simulink model "RefModel_AeroDyn_Sim2"  (R2019b)
settings: Solver=ode1  StartTime=tspan(1)  StopTime=inf  FixedStep=1/sensorFs.imuUpdateFs  RelTol=1e-3  EnableMultiTasking=on
undefined symbols (not defined in the file or in its folder): ACTUATOR_SET, Earth, ENVIRONMENT_SET, F, Light, MIL, sensorFs, SIM_SENSOR_SET, UAVPARAM_SET, WGS84
libraries: simulink x10, aerolibactuator x9, aerolibnav x6, sharedutil x5, shared6dofsys x3, aerolibwind2 x2, aerolibasang x2, aerolibatmos2 x1, aerolibconvert2 x1, aerolibgravity2 x1, aerolibtransform2 x1
(part 3 of 3)

== system RefModel_AeroDyn_Sim2/Sensor Model (noise)/Ublox1/add noise1 ==
  noise_flag : Inport
  signal : Inport  Port=2
  Add : Sum
  Add1 : Sum
  Divide : Product  Inputs=**
  Divide1 : Product  Inputs=**
  Divide2 : Product  Inputs=**
  MATLAB Function : MATLAB Function  TreatAsAtomicUnit=on
  Random Number : RandomNumber  Seed=[18,19,20]
  bias : Constant  Value=[0,0,0]
  bias1 : Constant  Value=SIM_SENSOR_SET.Ublox1.std_lla
  Out1 : Outport
  wires:
  bias1/1 -> Divide1/1
  bias/1 -> Add/1
  Divide/1 -> Add/2
  Random Number/1 -> Divide/1
  Divide1/1 -> Divide/2
  MATLAB Function/1(k) -> Divide1/2
  signal/1 -> MATLAB Function/1(u), Add1/2
  noise_flag/1 -> Divide2/1
  Divide2/1 -> Add1/1
  Add/1 -> Divide2/2
  Add1/1 -> Out1/1

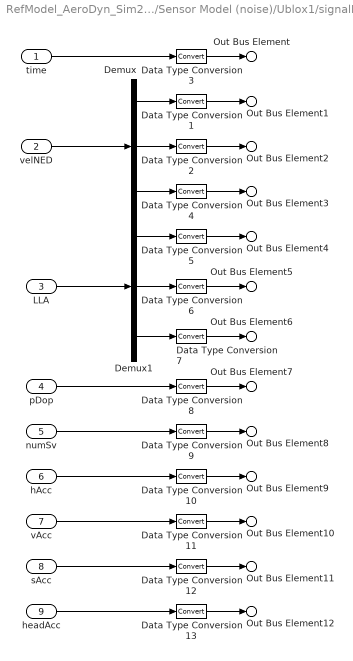
== system RefModel_AeroDyn_Sim2/Sensor Model (noise)/Ublox1/signalBus ==
  time : Inport
  velNED : Inport  Port=2
  LLA : Inport  Port=3
  pDop : Inport  Port=4
  numSv : Inport  Port=5
  hAcc : Inport  Port=6
  vAcc : Inport  Port=7
  sAcc : Inport  Port=8
  headAcc : Inport  Port=9
  Data Type Conversion{1..13} (13 alike) : DataTypeConversion
  Demux : Demux  Outputs=3
  Demux1 : Demux  Outputs=3
  Out Bus Element : Outport  PortName=bus  Element=time
  Out Bus Element1 : Outport  PortName=bus  Element=velN
  Out Bus Element2 : Outport  PortName=bus  Element=velE
  Out Bus Element3 : Outport  PortName=bus  Element=velD
  Out Bus Element4 : Outport  PortName=bus  Element=Lat
  Out Bus Element5 : Outport  PortName=bus  Element=Lon
  Out Bus Element6 : Outport  PortName=bus  Element=height
  Out Bus Element7 : Outport  PortName=bus  Element=pDop
  Out Bus Element8 : Outport  PortName=bus  Element=numSv
  Out Bus Element9 : Outport  PortName=bus  Element=hAcc
  Out Bus Element10 : Outport  PortName=bus  Element=vAcc
  Out Bus Element11 : Outport  PortName=bus  Element=sAcc
  Out Bus Element12 : Outport  PortName=bus  Element=headAcc
  wires:
  Demux/3 -> Data Type Conversion4/1
  Demux/2 -> Data Type Conversion2/1
  time/1 -> Data Type Conversion3/1
  Demux/1 -> Data Type Conversion1/1
  Demux1/1 -> Data Type Conversion5/1
  Demux1/2 -> Data Type Conversion6/1
  Demux1/3 -> Data Type Conversion7/1
  numSv/1 -> Data Type Conversion9/1
  pDop/1 -> Data Type Conversion8/1
  velNED/1 -> Demux/1
  LLA/1 -> Demux1/1
  Data Type Conversion3/1 -> Out Bus Element/1
  Data Type Conversion1/1 -> Out Bus Element1/1
  Data Type Conversion2/1 -> Out Bus Element2/1
  Data Type Conversion4/1 -> Out Bus Element3/1
  Data Type Conversion5/1 -> Out Bus Element4/1
  Data Type Conversion6/1 -> Out Bus Element5/1
  Data Type Conversion7/1 -> Out Bus Element6/1
  Data Type Conversion8/1 -> Out Bus Element7/1
  Data Type Conversion9/1 -> Out Bus Element8/1
  Data Type Conversion10/1 -> Out Bus Element9/1
  hAcc/1 -> Data Type Conversion10/1
  vAcc/1 -> Data Type Conversion11/1
  Data Type Conversion11/1 -> Out Bus Element10/1
  Data Type Conversion12/1 -> Out Bus Element11/1
  sAcc/1 -> Data Type Conversion12/1
  headAcc/1 -> Data Type Conversion13/1
  Data Type Conversion13/1 -> Out Bus Element12/1

== system RefModel_AeroDyn_Sim2/Sensor Model (noise)/um482/Subsystem ==
  Inport : Inport
  Inport1 : Inport  Port=2
  Demux7 : Demux  Outputs=3
  Demux8 : Demux  Outputs=3
  Mux : Mux  Inputs=2
  Mux1 : Mux  Inputs=2
  Mux2 : Mux  Inputs=2
  Outport : Outport
  Outport1 : Outport  Port=2
  Outport2 : Outport  Port=3
  wires:
  Demux7/1 -> Mux/1  "yaw [deg]"
  Demux8/1 -> Mux/2  "yaw [deg]"
  Inport/1 -> Demux7/1
  Mux/1 -> Outport/1
  Demux8/3 -> Mux2/2  "roll [deg]"
  Demux7/2 -> Mux1/1
  Inport1/1 -> Demux8/1
  Mux2/1 -> Outport2/1
  Mux1/1 -> Outport1/1
  Demux8/2 -> Mux1/2  "pitch [deg]"
  Demux7/3 -> Mux2/1  "roll [deg]"

== system RefModel_AeroDyn_Sim2/Sensor Model (noise)/um482/Subsystem1 ==
  Inport : Inport
  Inport1 : Inport  Port=2
  Demux7 : Demux  Outputs=3
  Demux8 : Demux  Outputs=3
  Mux : Mux  Inputs=2
  Mux1 : Mux  Inputs=2
  Mux2 : Mux  Inputs=2
  Outport : Outport
  Outport1 : Outport  Port=2
  Outport2 : Outport  Port=3
  wires:
  Demux7/3 -> Mux2/1  "roll [deg]"
  Demux8/2 -> Mux1/2  "pitch [deg]"
  Mux1/1 -> Outport1/1
  Mux2/1 -> Outport2/1
  Inport1/1 -> Demux8/1
  Demux7/2 -> Mux1/1
  Demux8/3 -> Mux2/2  "roll [deg]"
  Mux/1 -> Outport/1
  Inport/1 -> Demux7/1
  Demux8/1 -> Mux/2  "yaw [deg]"
  Demux7/1 -> Mux/1  "yaw [deg]"

== system RefModel_AeroDyn_Sim2/Sensor Model (noise)/um482/Subsystem2 ==
  In : Inport
  Compare To Zero : simulink/Logic and Bit Operations/Compare To Zero  relop===  OutDataTypeStr=boolean
  Constant : Constant  Value=1/sample_freq
  Digital Clock : DigitalClock  SampleTime=1/sensorFs.imuUpdateFs
  Math Function : Math  Operator=rem  SignedPower=off  SaturateOnIntegerOverflow=on
  Scope1 : Scope
  Subsystem : Subsystem
  zeroHold : Outport
  wires:
  Digital Clock/1 -> Math Function/1
  Constant/1 -> Math Function/2
  Math Function/1 -> Compare To Zero/1
  Compare To Zero/1 -> Scope1/1, Subsystem/Enable
  Subsystem/1(Out1) -> zeroHold/1
  In/1 -> Subsystem/1(In1)

== system RefModel_AeroDyn_Sim2/Sensor Model (noise)/um482/add noise ==
  noise_flag : Inport
  signal : Inport  Port=2
  Add : Sum
  Add1 : Sum
  Divide : Product  Inputs=**
  Divide1 : Product  Inputs=**
  Random Number : RandomNumber  Seed=[18,19,20]
  bias : Constant  Value=[0,0,0]
  bias1 : Constant  Value=SIM_SENSOR_SET.um482.std_gpsvel
  Out1 : Outport
  wires:
  signal/1 -> Add1/2
  Random Number/1 -> Divide/1
  Divide/1 -> Add/2
  bias/1 -> Add/1
  bias1/1 -> Divide/2
  Add/1 -> Divide1/2
  Divide1/1 -> Add1/1
  noise_flag/1 -> Divide1/1
  Add1/1 -> Out1/1

== system RefModel_AeroDyn_Sim2/Sensor Model (noise)/um482/add noise1 ==
  noise_flag : Inport
  signal : Inport  Port=2
  Add : Sum
  Add1 : Sum
  Divide : Product  Inputs=**
  Divide1 : Product  Inputs=**
  Divide2 : Product  Inputs=**
  MATLAB Function : MATLAB Function  TreatAsAtomicUnit=on
  Random Number : RandomNumber  Seed=[18,19,20]
  bias : Constant  Value=[0,0,0]
  bias1 : Constant  Value=SIM_SENSOR_SET.um482.std_lla
  Out1 : Outport
  wires:
  bias1/1 -> Divide1/1
  bias/1 -> Add/1
  Divide/1 -> Add/2
  Random Number/1 -> Divide/1
  Divide1/1 -> Divide/2
  MATLAB Function/1(k) -> Divide1/2
  signal/1 -> MATLAB Function/1(u), Add1/2
  noise_flag/1 -> Divide2/1
  Divide2/1 -> Add1/1
  Add/1 -> Divide2/2
  Add1/1 -> Out1/1

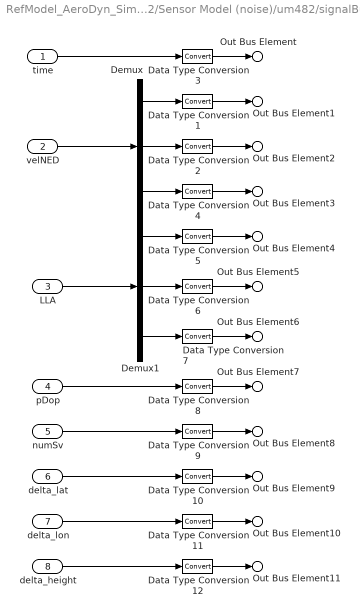
== system RefModel_AeroDyn_Sim2/Sensor Model (noise)/um482/signalBus ==
  time : Inport
  velNED : Inport  Port=2
  LLA : Inport  Port=3
  pDop : Inport  Port=4
  numSv : Inport  Port=5
  delta_lat : Inport  Port=6
  delta_lon : Inport  Port=7
  delta_height : Inport  Port=8
  Data Type Conversion{1..12} (12 alike) : DataTypeConversion
  Demux : Demux  Outputs=3
  Demux1 : Demux  Outputs=3
  Out Bus Element : Outport  PortName=bus  Element=time
  Out Bus Element1 : Outport  PortName=bus  Element=velN
  Out Bus Element2 : Outport  PortName=bus  Element=velE
  Out Bus Element3 : Outport  PortName=bus  Element=velD
  Out Bus Element4 : Outport  PortName=bus  Element=Lat
  Out Bus Element5 : Outport  PortName=bus  Element=Lon
  Out Bus Element6 : Outport  PortName=bus  Element=height
  Out Bus Element7 : Outport  PortName=bus  Element=pDop
  Out Bus Element8 : Outport  PortName=bus  Element=numSv
  Out Bus Element9 : Outport  PortName=bus  Element=delta_lat
  Out Bus Element10 : Outport  PortName=bus  Element=delta_lon
  Out Bus Element11 : Outport  PortName=bus  Element=delta_height
  wires:
  Demux/3 -> Data Type Conversion4/1
  Demux/2 -> Data Type Conversion2/1
  time/1 -> Data Type Conversion3/1
  Demux/1 -> Data Type Conversion1/1
  Demux1/1 -> Data Type Conversion5/1
  Demux1/2 -> Data Type Conversion6/1
  Demux1/3 -> Data Type Conversion7/1
  numSv/1 -> Data Type Conversion9/1
  pDop/1 -> Data Type Conversion8/1
  velNED/1 -> Demux/1
  LLA/1 -> Demux1/1
  Data Type Conversion3/1 -> Out Bus Element/1
  Data Type Conversion1/1 -> Out Bus Element1/1
  Data Type Conversion2/1 -> Out Bus Element2/1
  Data Type Conversion4/1 -> Out Bus Element3/1
  Data Type Conversion5/1 -> Out Bus Element4/1
  Data Type Conversion6/1 -> Out Bus Element5/1
  Data Type Conversion7/1 -> Out Bus Element6/1
  Data Type Conversion8/1 -> Out Bus Element7/1
  Data Type Conversion9/1 -> Out Bus Element8/1
  Data Type Conversion10/1 -> Out Bus Element9/1
  delta_lat/1 -> Data Type Conversion10/1
  delta_lon/1 -> Data Type Conversion11/1
  Data Type Conversion11/1 -> Out Bus Element10/1
  Data Type Conversion12/1 -> Out Bus Element11/1
  delta_height/1 -> Data Type Conversion12/1

== system RefModel_AeroDyn_Sim2/UAV Dynamics/6DOF (Quaternion)/Velocity Conversion ==
  in : Inport  Unit=m/s
  Unit Conversion : UnitConversion
  out : Outport  VectorParamsAs1DForOutWhenUnconnected=off
  wires:
  Unit Conversion/1 -> out/1
  in/1 -> Unit Conversion/1

== system RefModel_AeroDyn_Sim2/UAV Dynamics/6DOF (Quaternion)/Velocity Conversion1 ==
  in : Inport  Unit=m/s
  Unit Conversion : UnitConversion
  out : Outport  VectorParamsAs1DForOutWhenUnconnected=off
  wires:
  Unit Conversion/1 -> out/1
  in/1 -> Unit Conversion/1

== system RefModel_AeroDyn_Sim2/UAV Dynamics/6DOF (Quaternion)/Velocity Conversion2 ==
  in : Inport  Unit=m/s
  Unit Conversion : UnitConversion
  out : Outport  Unit=m/s  VectorParamsAs1DForOutWhenUnconnected=off
  wires:
  Unit Conversion/1 -> out/1
  in/1 -> Unit Conversion/1

== system RefModel_AeroDyn_Sim2/UAV Dynamics/6DOF (Quaternion)/transform to Inertial axes  ==
  x y z : Inport
  transform coefficients : Inport  Port=2
  Product : Product  Multiplication=Matrix(*)  SaturateOnIntegerOverflow=on  InputSameDT=on  OutDataTypeStr=Inherit: Same as first input
  Reshape1 : Reshape  OutputDimensionality=Column vector (2-D)
  Reshape2 : Reshape
  Ve : Outport  VectorParamsAs1DForOutWhenUnconnected=off
  wires:
  Reshape2/1 -> Ve/1
  Reshape1/1 -> Product/2
  x y z/1 -> Reshape1/1
  transform coefficients/1 -> Product/1
  Product/1 -> Reshape2/1

== system RefModel_AeroDyn_Sim2/Force and Moment/Aero Surface/Lateral Channel/CY ==
  beta : Inport
  rudder : Inport  Port=2
  airspeed : Inport  Port=3
  CYDr : Constant  Value=UAVPARAM_SET.AeroParam.CY_rudder
      settings: AttributesFormatString=%<Value>
  CYb : Constant  Value=UAVPARAM_SET.AeroParam.CY_beta
      settings: AttributesFormatString=%<Value>
  Product : Product  SaturateOnIntegerOverflow=on  OutDataTypeStr=Inherit: Same as first input
  Product1 : Product  SaturateOnIntegerOverflow=on  OutDataTypeStr=Inherit: Same as first input
  Sum2 : Sum  SaturateOnIntegerOverflow=on
  CY : Outport  VectorParamsAs1DForOutWhenUnconnected=off
  wires:
  Product1/1 -> Sum2/2
  rudder/1 -> Product1/2
  CYDr/1 -> Product1/1
  Product/1 -> Sum2/1
  Sum2/1 -> CY/1
  beta/1 -> Product/2
  CYb/1 -> Product/1

== system RefModel_AeroDyn_Sim2/Force and Moment/Aero Surface/Lateral Channel/Cl ==
  beta : Inport
  aileron : Inport  Port=2
  rudder : Inport  Port=3
  p,q,r : Inport  Port=4
  Airspeed : Inport  Port=5
  wingspan : Inport  Port=6
  ClDa : Constant  Value=UAVPARAM_SET.AeroParam.Cl_aileron
      settings: AttributesFormatString=%<Value>
  ClDr : Constant  Value=UAVPARAM_SET.AeroParam.Cl_rudder
      settings: AttributesFormatString=%<Value>
  Clb : Constant  Value=UAVPARAM_SET.AeroParam.Cl_beta
      settings: AttributesFormatString=%<Value>
  Product1 : Product  SaturateOnIntegerOverflow=on  OutDataTypeStr=Inherit: Same as first input
  Product4 : Product  SaturateOnIntegerOverflow=on  OutDataTypeStr=Inherit: Same as first input
  Product5 : Product  SaturateOnIntegerOverflow=on  OutDataTypeStr=Inherit: Same as first input
  Sum : Sum  Inputs=+++++  SaturateOnIntegerOverflow=on
  roll factors : Subsystem
  Cl : Outport  VectorParamsAs1DForOutWhenUnconnected=off
  wires:
  roll factors/1(Clp) -> Sum/4
  Product5/1 -> Sum/2  "CldA"
  Airspeed/1 -> roll factors/2(Airspeed)
  p,q,r/1 -> roll factors/1(p,q,r)
  roll factors/2(Clr) -> Sum/5
  Product1/1 -> Sum/3  "Cldr"
  Product4/1 -> Sum/1  "Clb"
  Sum/1 -> Cl/1
  rudder/1 -> Product1/2
  ClDr/1 -> Product1/1
  aileron/1 -> Product5/2
  ClDa/1 -> Product5/1
  beta/1 -> Product4/2
  Clb/1 -> Product4/1
  wingspan/1 -> roll factors/3(wingspan)

== system RefModel_AeroDyn_Sim2/Force and Moment/Aero Surface/Lateral Channel/Cn ==
  beta : Inport
  aileron : Inport  Port=2
  rudder : Inport  Port=3
  p,q,r : Inport  Port=4
  Airspeed : Inport  Port=5
  wingspan : Inport  Port=6
  CnDa : Constant  Value=UAVPARAM_SET.AeroParam.Cn_aileron
      settings: AttributesFormatString=%<Value>
  CnDr : Constant  Value=UAVPARAM_SET.AeroParam.Cn_rudder
      settings: AttributesFormatString=%<Value>
  Cnb : Constant  Value=UAVPARAM_SET.AeroParam.Cn_beta
      settings: AttributesFormatString=%<Value>
  Product1 : Product  SaturateOnIntegerOverflow=on  OutDataTypeStr=Inherit: Same as first input
  Product4 : Product  SaturateOnIntegerOverflow=on  OutDataTypeStr=Inherit: Same as first input
  Product5 : Product  SaturateOnIntegerOverflow=on  OutDataTypeStr=Inherit: Same as first input
  Sum : Sum  Inputs=+++++  SaturateOnIntegerOverflow=on
  yaw factors : Subsystem
  Cn : Outport  VectorParamsAs1DForOutWhenUnconnected=off
  wires:
  Airspeed/1 -> yaw factors/2(Airspeed)
  p,q,r/1 -> yaw factors/1(p,q,r)
  Cnb/1 -> Product4/1
  beta/1 -> Product4/2
  CnDa/1 -> Product5/1
  Product5/1 -> Sum/2
  aileron/1 -> Product5/2
  CnDr/1 -> Product1/1
  rudder/1 -> Product1/2
  Sum/1 -> Cn/1
  Product1/1 -> Sum/3
  yaw factors/2(Cnr) -> Sum/5
  yaw factors/1(Cnp) -> Sum/4
  Product4/1 -> Sum/1
  wingspan/1 -> yaw factors/3(wingspan)

== system RefModel_AeroDyn_Sim2/Force and Moment/Aero Surface/Longitudinal Channel/CD ==
  alpha : Inport
  airspeed : Inport  Port=2
  Apolar (A2) : Constant  Value=UAVPARAM_SET.AeroParam.CD_alpha
      settings: AttributesFormatString=%<Value>
  CD0 : Constant  Value=UAVPARAM_SET.AeroParam.CD0
      settings: AttributesFormatString=%<Value>
  Gain : Gain  Gain=-1  SaturateOnIntegerOverflow=on  OutDataTypeStr=Inherit: Same as input  ParamDataTypeStr=Inherit: Same as input
      settings: AttributesFormatString=%<Gain>
  Product : Product  SaturateOnIntegerOverflow=on  OutDataTypeStr=Inherit: Same as first input
  Sum1 : Sum  Inputs=|++  SaturateOnIntegerOverflow=on
  CD : Outport  VectorParamsAs1DForOutWhenUnconnected=off
  wires:
  Gain/1 -> CD/1
  Apolar (A2)/1 -> Product/1
  alpha/1 -> Product/2
  Sum1/1 -> Gain/1
  Product/1 -> Sum1/1
  CD0/1 -> Sum1/2

== system RefModel_AeroDyn_Sim2/Force and Moment/Aero Surface/Longitudinal Channel/CL ==
  alpha : Inport
  elevator : Inport  Port=2
  airspeed : Inport  Port=3
  CL0 : Constant  Value=UAVPARAM_SET.AeroParam.CL0
      settings: AttributesFormatString=%<Value>
  CLDe : Constant  Value=UAVPARAM_SET.AeroParam.CL_elevator
      settings: AttributesFormatString=%<Value>
  CLa : Constant  Value=UAVPARAM_SET.AeroParam.CL_alpha
      settings: AttributesFormatString=%<Value>
  Product1 : Product  SaturateOnIntegerOverflow=on  OutDataTypeStr=Inherit: Same as first input
  Product4 : Product  SaturateOnIntegerOverflow=on  OutDataTypeStr=Inherit: Same as first input
  Sum : Sum  Inputs=++++  SaturateOnIntegerOverflow=on
  Y-down : Gain  Gain=-1  SaturateOnIntegerOverflow=on  OutDataTypeStr=Inherit: Same as input  ParamDataTypeStr=Inherit: Same as input
      settings: AttributesFormatString=%<Gain>
  CL : Outport  VectorParamsAs1DForOutWhenUnconnected=off
  wires:
  CL0/1 -> Sum/1
  Product1/1 -> Sum/3
  Sum/1 -> Y-down/1
  elevator/1 -> Product1/2
  CLDe/1 -> Product1/1
  alpha/1 -> Product4/2
  CLa/1 -> Product4/1
  Product4/1 -> Sum/2
  Y-down/1 -> CL/1  "CL"

== system RefModel_AeroDyn_Sim2/Force and Moment/Aero Surface/Longitudinal Channel/Cm ==
  alpha : Inport
  De : Inport  Port=2
  p,q,r : Inport  Port=3
  airspeed : Inport  Port=4
  Cm0 : Constant  Value=UAVPARAM_SET.AeroParam.Cm0
      settings: AttributesFormatString=%<Value>
  CmDe : Constant  Value=UAVPARAM_SET.AeroParam.Cm_elevator
      settings: AttributesFormatString=%<Value>
  Cma : Constant  Value=UAVPARAM_SET.AeroParam.Cm_alpha
      settings: AttributesFormatString=%<Value>
  Cma1 : Constant  Value=UAVPARAM_SET.AeroParam.Cm_q
      settings: AttributesFormatString=%<Value>
  Get q : Selector  InputPortWidth=3  IndexOptions=Index vector (dialog)  Indices=2  OutputSizes=[(-2)]
  Product1 : Product  SaturateOnIntegerOverflow=on  OutDataTypeStr=Inherit: Same as first input
  Product3 : Product  SaturateOnIntegerOverflow=on  OutDataTypeStr=Inherit: Same as first input
  Product4 : Product  SaturateOnIntegerOverflow=on  OutDataTypeStr=Inherit: Same as first input
  Sum : Sum  Inputs=+++++  SaturateOnIntegerOverflow=on
  Cm : Outport  VectorParamsAs1DForOutWhenUnconnected=off
  wires:
  Get q/1 -> Product3/2
  Product3/1 -> Sum/5  "cmq"
  p,q,r/1 -> Get q/1
  Cma1/1 -> Product3/1
  Product1/1 -> Sum/3  "cmde"
  Product4/1 -> Sum/2  "cma"
  Sum/1 -> Cm/1  "total"
  De/1 -> Product1/2
  CmDe/1 -> Product1/1
  alpha/1 -> Product4/2
  Cma/1 -> Product4/1
  Cm0/1 -> Sum/1  "cm0"

== system RefModel_AeroDyn_Sim2/Force and Moment/Rotor Force/Left Back/Rotor 2814 ==
  pwm : Inport
  Constant : Constant  Value=ACTUATOR_SET.tiltRotor.poly_fromPwmTopull
  Constant1 : Constant  Value=ACTUATOR_SET.tiltRotor.poly_fromPwmToTorque
  Constant2 : Constant  Value=[0,0]
  Constant3 : Constant  Value=ACTUATOR_SET.tiltRotorLeft.torqueSign
  Divide : Product  Inputs=**
  MATLAB Function : MATLAB Function  TreatAsAtomicUnit=on
  MATLAB Function1 : MATLAB Function  TreatAsAtomicUnit=on
  Mux : Mux  Inputs=2
  pull : Outport
  torque : Outport  Port=2
  wires:
  pwm/1 -> MATLAB Function1/1(u), MATLAB Function/1(u)
  MATLAB Function/1(y) -> pull/1
  Constant/1 -> MATLAB Function/2(poly)
  Constant1/1 -> MATLAB Function1/2(poly)
  MATLAB Function1/1(y) -> Divide/1
  Constant3/1 -> Divide/2
  Divide/1 -> Mux/2
  Constant2/1 -> Mux/1
  Mux/1 -> torque/1

== system RefModel_AeroDyn_Sim2/Force and Moment/Rotor Force/Left Forward/Rotor 5208 ==
  pwm : Inport
  Constant : Constant  Value=ACTUATOR_SET.verticalRotor.poly_fromPwmTopull
  Constant1 : Constant  Value=ACTUATOR_SET.verticalRotor.poly_fromPwmToTorque
  Constant2 : Constant  Value=[0,0]
  Constant3 : Constant  Value=ACTUATOR_SET.verticalRotorLeft.torqueSign
  Divide : Product  Inputs=**
  MATLAB Function : MATLAB Function  TreatAsAtomicUnit=on
  MATLAB Function1 : MATLAB Function  TreatAsAtomicUnit=on
  Mux : Mux  Inputs=2
  pull : Outport
  torque : Outport  Port=2
  wires:
  Constant1/1 -> MATLAB Function1/2(poly)
  Constant/1 -> MATLAB Function/2(poly)
  MATLAB Function/1(y) -> pull/1
  pwm/1 -> MATLAB Function/1(u), MATLAB Function1/1(u)
  Constant2/1 -> Mux/1
  Mux/1 -> torque/1
  Constant3/1 -> Divide/2
  MATLAB Function1/1(y) -> Divide/1
  Divide/1 -> Mux/2

== system RefModel_AeroDyn_Sim2/Force and Moment/Rotor Force/Right Back/Rotor 2814 ==
  pwm : Inport
  Constant : Constant  Value=ACTUATOR_SET.tiltRotor.poly_fromPwmTopull
  Constant1 : Constant  Value=ACTUATOR_SET.tiltRotor.poly_fromPwmToTorque
  Constant2 : Constant  Value=[0,0]
  Constant3 : Constant  Value=ACTUATOR_SET.tiltRotorRight.torqueSign
  Divide : Product  Inputs=**
  MATLAB Function : MATLAB Function  TreatAsAtomicUnit=on
  MATLAB Function1 : MATLAB Function  TreatAsAtomicUnit=on
  Mux : Mux  Inputs=2
  pull : Outport
  torque : Outport  Port=2
  wires:
  pwm/1 -> MATLAB Function1/1(u), MATLAB Function/1(u)
  MATLAB Function/1(y) -> pull/1
  Constant/1 -> MATLAB Function/2(poly)
  Constant1/1 -> MATLAB Function1/2(poly)
  Constant2/1 -> Mux/1
  Constant3/1 -> Divide/2
  Divide/1 -> Mux/2
  Mux/1 -> torque/1
  MATLAB Function1/1(y) -> Divide/1

== system RefModel_AeroDyn_Sim2/Force and Moment/Rotor Force/Right Forward/Rotor 5208 ==
  pwm : Inport
  Constant : Constant  Value=ACTUATOR_SET.verticalRotor.poly_fromPwmTopull
  Constant1 : Constant  Value=ACTUATOR_SET.verticalRotor.poly_fromPwmToTorque
  Constant2 : Constant  Value=[0,0]
  Constant3 : Constant  Value=ACTUATOR_SET.verticalRotorRight.torqueSign
  Divide : Product  Inputs=**
  MATLAB Function : MATLAB Function  TreatAsAtomicUnit=on
  MATLAB Function1 : MATLAB Function  TreatAsAtomicUnit=on
  Mux : Mux  Inputs=2
  pull : Outport
  torque : Outport  Port=2
  wires:
  Constant1/1 -> MATLAB Function1/2(poly)
  Constant/1 -> MATLAB Function/2(poly)
  MATLAB Function/1(y) -> pull/1
  pwm/1 -> MATLAB Function1/1(u), MATLAB Function/1(u)
  Constant2/1 -> Mux/1
  Mux/1 -> torque/1
  MATLAB Function1/1(y) -> Divide/1
  Divide/1 -> Mux/2
  Constant3/1 -> Divide/2

== system RefModel_AeroDyn_Sim2/Sensor Model (noise)/Airspeed1/Subsystem3/Subsystem ==
  In1 : Inport
  Enable : EnablePort
  Out1 : Outport
  wires:
  In1/1 -> Out1/1

== system RefModel_AeroDyn_Sim2/Sensor Model (noise)/Baro1/Subsystem3/Subsystem ==
  In1 : Inport
  Enable : EnablePort
  Out1 : Outport
  wires:
  In1/1 -> Out1/1

== system RefModel_AeroDyn_Sim2/Sensor Model (noise)/IMU1/Subsystem2/Subsystem ==
  In1 : Inport
  Enable : EnablePort
  Out1 : Outport
  wires:
  In1/1 -> Out1/1

== system RefModel_AeroDyn_Sim2/Sensor Model (noise)/IMU1/Subsystem3/NOISE ==
  In1 : Inport
  In2 : Inport  Port=2
  In3 : Inport  Port=3
  In4 : Inport  Port=4
  In5 : Inport  Port=5
  Action Port : ActionPort  ActionPortLabel=case [ 1 ]:
  Three-axis Inertial Measurement Unit : aerolibnav/Three-axis Inertial Measurement Unit  units=Metric (MKS)  imu=[0 0 0]  i_Ts=1/sensorFs.imuUpdateFs  dtype_a=off  w_a=190  z_a=0.707  a_sf_cc=[1 0 0; 0 1 0; 0 0 1]  a_bias=SIM_SENSOR_SET.IMU1.acc_bias  a_sat="[-inf  -inf  -inf  inf inf inf]"  dtype_g=off  w_g=190  z_g=0.707  g_sf_cc=[1 0 0; 0 1 0; 0 0 1]  g_bias=SIM_SENSOR_SET.IMU1.gyro_bias  g_sens=[0 0 0]  g_sat="[-inf  -inf  -inf  inf inf inf]"  i_rand=on  i_seeds=[23093 23094 23095 23096 23097 23098]  i_pow=[SIM_SENSOR_SET.IMU1.S_acc, SIM_SENSOR_SET.IMU1.S_gyro]
  accel : Outport
  Out2 : Outport  Port=2
  wires:
  In1/1 -> Three-axis Inertial Measurement Unit/1
  In2/1 -> Three-axis Inertial Measurement Unit/2
  Three-axis Inertial Measurement Unit/2 -> Out2/1
  Three-axis Inertial Measurement Unit/1 -> accel/1  "accel"
  In5/1 -> Three-axis Inertial Measurement Unit/5
  In3/1 -> Three-axis Inertial Measurement Unit/3
  In4/1 -> Three-axis Inertial Measurement Unit/4

== system RefModel_AeroDyn_Sim2/Sensor Model (noise)/IMU1/Subsystem3/NOISE FREE ==
  In1 : Inport
  In2 : Inport  Port=2
  In3 : Inport  Port=3
  In4 : Inport  Port=4
  In5 : Inport  Port=5
  Action Port : ActionPort  ActionPortLabel=default:
  Three-axis Inertial Measurement Unit1 : aerolibnav/Three-axis Inertial Measurement Unit  units=Metric (MKS)  imu=[0 0 0]  i_Ts=1/sensorFs.imuUpdateFs  dtype_a=off  w_a=190  z_a=0.707  a_sf_cc=[1 0 0; 0 1 0; 0 0 1]  a_bias=[0,0,0]  a_sat="[-inf  -inf  -inf  inf inf inf]"  dtype_g=off  w_g=190  z_g=0.707  g_sf_cc=[1 0 0; 0 1 0; 0 0 1]  g_bias=[0 0 0]  g_sens=[0 0 0]  g_sat="[-inf  -inf  -inf  inf inf inf]"  i_rand=off  i_seeds=[23093 23094 23095 23096 23097 23098]  i_pow=[SIM_SENSOR_SET.IMU1.S_acc, SIM_SENSOR_SET.IMU1.S_gyro]
  accel : Outport
  Out2 : Outport  Port=2
  wires:
  In2/1 -> Three-axis Inertial Measurement Unit1/2
  In1/1 -> Three-axis Inertial Measurement Unit1/1
  In5/1 -> Three-axis Inertial Measurement Unit1/5
  Three-axis Inertial Measurement Unit1/1 -> accel/1  "accel"
  In3/1 -> Three-axis Inertial Measurement Unit1/3
  In4/1 -> Three-axis Inertial Measurement Unit1/4
  Three-axis Inertial Measurement Unit1/2 -> Out2/1

== system RefModel_AeroDyn_Sim2/Sensor Model (noise)/IMU2/Subsystem2/Subsystem ==
  In1 : Inport
  Enable : EnablePort
  Out1 : Outport
  wires:
  In1/1 -> Out1/1

== system RefModel_AeroDyn_Sim2/Sensor Model (noise)/IMU2/Subsystem3/NOISE ==
  In1 : Inport
  In2 : Inport  Port=2
  In3 : Inport  Port=3
  In4 : Inport  Port=4
  In5 : Inport  Port=5
  Action Port : ActionPort  ActionPortLabel=case [ 1 ]:
  Three-axis Inertial Measurement Unit : aerolibnav/Three-axis Inertial Measurement Unit  units=Metric (MKS)  imu=[0 0 0]  i_Ts=1/sensorFs.imuUpdateFs  dtype_a=off  w_a=190  z_a=0.707  a_sf_cc=[1 0 0; 0 1 0; 0 0 1]  a_bias=SIM_SENSOR_SET.IMU2.acc_bias  a_sat="[-inf  -inf  -inf  inf inf inf]"  dtype_g=off  w_g=190  z_g=0.707  g_sf_cc=[1 0 0; 0 1 0; 0 0 1]  g_bias=SIM_SENSOR_SET.IMU2.gyro_bias  g_sens=[0 0 0]  g_sat="[-inf  -inf  -inf  inf inf inf]"  i_rand=on  i_seeds=[23093 23094 23095 23096 23097 23098]  i_pow=[SIM_SENSOR_SET.IMU2.S_acc, SIM_SENSOR_SET.IMU2.S_gyro]
  accel : Outport
  Out2 : Outport  Port=2
  wires:
  In1/1 -> Three-axis Inertial Measurement Unit/1
  In2/1 -> Three-axis Inertial Measurement Unit/2
  Three-axis Inertial Measurement Unit/2 -> Out2/1
  Three-axis Inertial Measurement Unit/1 -> accel/1  "accel"
  In5/1 -> Three-axis Inertial Measurement Unit/5
  In3/1 -> Three-axis Inertial Measurement Unit/3
  In4/1 -> Three-axis Inertial Measurement Unit/4

== system RefModel_AeroDyn_Sim2/Sensor Model (noise)/IMU2/Subsystem3/NOISE FREE ==
  In1 : Inport
  In2 : Inport  Port=2
  In3 : Inport  Port=3
  In4 : Inport  Port=4
  In5 : Inport  Port=5
  Action Port : ActionPort  ActionPortLabel=default:
  Three-axis Inertial Measurement Unit1 : aerolibnav/Three-axis Inertial Measurement Unit  units=Metric (MKS)  imu=[0 0 0]  i_Ts=1/sensorFs.imuUpdateFs  dtype_a=off  w_a=190  z_a=0.707  a_sf_cc=[1 0 0; 0 1 0; 0 0 1]  a_bias=[0,0,0]  a_sat="[-inf  -inf  -inf  inf inf inf]"  dtype_g=off  w_g=190  z_g=0.707  g_sf_cc=[1 0 0; 0 1 0; 0 0 1]  g_bias=[0 0 0]  g_sens=[0 0 0]  g_sat="[-inf  -inf  -inf  inf inf inf]"  i_rand=off  i_seeds=[23093 23094 23095 23096 23097 23098]  i_pow=[SIM_SENSOR_SET.IMU1.S_acc, SIM_SENSOR_SET.IMU1.S_gyro]
  accel : Outport
  Out2 : Outport  Port=2
  wires:
  In2/1 -> Three-axis Inertial Measurement Unit1/2
  In1/1 -> Three-axis Inertial Measurement Unit1/1
  In5/1 -> Three-axis Inertial Measurement Unit1/5
  Three-axis Inertial Measurement Unit1/1 -> accel/1  "accel"
  In3/1 -> Three-axis Inertial Measurement Unit1/3
  In4/1 -> Three-axis Inertial Measurement Unit1/4
  Three-axis Inertial Measurement Unit1/2 -> Out2/1

== system RefModel_AeroDyn_Sim2/Sensor Model (noise)/IMU3/Subsystem2/Subsystem ==
  In1 : Inport
  Enable : EnablePort
  Out1 : Outport
  wires:
  In1/1 -> Out1/1

== system RefModel_AeroDyn_Sim2/Sensor Model (noise)/IMU3/Subsystem3/NOISE ==
  In1 : Inport
  In2 : Inport  Port=2
  In3 : Inport  Port=3
  In4 : Inport  Port=4
  In5 : Inport  Port=5
  Action Port : ActionPort  ActionPortLabel=case [ 1 ]:
  Three-axis Inertial Measurement Unit : aerolibnav/Three-axis Inertial Measurement Unit  units=Metric (MKS)  imu=[0 0 0]  i_Ts=1/sensorFs.imuUpdateFs  dtype_a=off  w_a=190  z_a=0.707  a_sf_cc=[1 0 0; 0 1 0; 0 0 1]  a_bias=SIM_SENSOR_SET.IMU3.acc_bias  a_sat="[-inf  -inf  -inf  inf inf inf]"  dtype_g=off  w_g=190  z_g=0.707  g_sf_cc=[1 0 0; 0 1 0; 0 0 1]  g_bias=SIM_SENSOR_SET.IMU3.gyro_bias  g_sens=[0 0 0]  g_sat="[-inf  -inf  -inf  inf inf inf]"  i_rand=on  i_seeds=[23093 23094 23095 23096 23097 23098]  i_pow=[SIM_SENSOR_SET.IMU3.S_acc, SIM_SENSOR_SET.IMU3.S_gyro]
  accel : Outport
  Out2 : Outport  Port=2
  wires:
  In4/1 -> Three-axis Inertial Measurement Unit/4
  In3/1 -> Three-axis Inertial Measurement Unit/3
  In5/1 -> Three-axis Inertial Measurement Unit/5
  Three-axis Inertial Measurement Unit/1 -> accel/1  "accel"
  Three-axis Inertial Measurement Unit/2 -> Out2/1
  In2/1 -> Three-axis Inertial Measurement Unit/2
  In1/1 -> Three-axis Inertial Measurement Unit/1

== system RefModel_AeroDyn_Sim2/Sensor Model (noise)/IMU3/Subsystem3/NOISE FREE ==
  In1 : Inport
  In2 : Inport  Port=2
  In3 : Inport  Port=3
  In4 : Inport  Port=4
  In5 : Inport  Port=5
  Action Port : ActionPort  ActionPortLabel=default:
  Three-axis Inertial Measurement Unit1 : aerolibnav/Three-axis Inertial Measurement Unit  units=Metric (MKS)  imu=[0 0 0]  i_Ts=1/sensorFs.imuUpdateFs  dtype_a=off  w_a=190  z_a=0.707  a_sf_cc=[1 0 0; 0 1 0; 0 0 1]  a_bias=[0,0,0]  a_sat="[-inf  -inf  -inf  inf inf inf]"  dtype_g=off  w_g=190  z_g=0.707  g_sf_cc=[1 0 0; 0 1 0; 0 0 1]  g_bias=[0 0 0]  g_sens=[0 0 0]  g_sat="[-inf  -inf  -inf  inf inf inf]"  i_rand=off  i_seeds=[23093 23094 23095 23096 23097 23098]  i_pow=[SIM_SENSOR_SET.IMU1.S_acc, SIM_SENSOR_SET.IMU1.S_gyro]
  accel : Outport
  Out2 : Outport  Port=2
  wires:
  In2/1 -> Three-axis Inertial Measurement Unit1/2
  In1/1 -> Three-axis Inertial Measurement Unit1/1
  In5/1 -> Three-axis Inertial Measurement Unit1/5
  Three-axis Inertial Measurement Unit1/1 -> accel/1  "accel"
  In3/1 -> Three-axis Inertial Measurement Unit1/3
  In4/1 -> Three-axis Inertial Measurement Unit1/4
  Three-axis Inertial Measurement Unit1/2 -> Out2/1

== system RefModel_AeroDyn_Sim2/Sensor Model (noise)/Mag1/Subsystem9/Subsystem ==
  In1 : Inport
  Enable : EnablePort
  Out1 : Outport
  wires:
  In1/1 -> Out1/1

== system RefModel_AeroDyn_Sim2/Sensor Model (noise)/Mag2/Subsystem9/Subsystem ==
  In1 : Inport
  Enable : EnablePort
  Out1 : Outport
  wires:
  In1/1 -> Out1/1

== system RefModel_AeroDyn_Sim2/Sensor Model (noise)/Radar1/Subsystem3/Subsystem ==
  In1 : Inport
  Enable : EnablePort
  Out1 : Outport
  wires:
  In1/1 -> Out1/1

== system RefModel_AeroDyn_Sim2/Sensor Model (noise)/Ublox1/Subsystem2/Subsystem ==
  In1 : Inport
  Enable : EnablePort
  Out1 : Outport
  wires:
  In1/1 -> Out1/1

== system RefModel_AeroDyn_Sim2/Sensor Model (noise)/um482/Subsystem2/Subsystem ==
  In1 : Inport
  Enable : EnablePort
  Out1 : Outport
  wires:
  In1/1 -> Out1/1

== system RefModel_AeroDyn_Sim2/Force and Moment/Aero Surface/Lateral Channel/Cl/roll factors ==
  p,q,r : Inport
  Airspeed : Inport  Port=2
  wingspan : Inport  Port=3
  Constant : Constant  Value=UAVPARAM_SET.AeroParam.Cl_p
      settings: AttributesFormatString=%<Value>
  Constant1 : Constant  Value=UAVPARAM_SET.AeroParam.Cl_r
      settings: AttributesFormatString=%<Value>
  Get p : Selector  InputPortWidth=3  IndexOptions=Index vector (dialog)  Indices=1  OutputSizes=[(-2)]
  Get r : Selector  InputPortWidth=3  IndexOptions=Index vector (dialog)  Indices=3  OutputSizes=[(-2)]
  Product : Product  SaturateOnIntegerOverflow=on  OutDataTypeStr=Inherit: Same as first input
  Product1 : Product  SaturateOnIntegerOverflow=on  OutDataTypeStr=Inherit: Same as first input
  roll rate fact : Subsystem
  yaw rate fact : Subsystem  AncestorBlock=mbdriLib/Utilities/yaw rate fact
  Clp : Outport  VectorParamsAs1DForOutWhenUnconnected=off
  Clr : Outport  Port=2  VectorParamsAs1DForOutWhenUnconnected=off
  wires:
  Get r/1 -> yaw rate fact/1(r)
  p,q,r/1 -> Get r/1, Get p/1
  Get p/1 -> roll rate fact/1(p)
  Airspeed/1 -> roll rate fact/2(Airspeed), yaw rate fact/2(Airspeed)
  yaw rate fact/1(Yaw Rate Fac) -> Product1/2
  Constant1/1 -> Product1/1
  roll rate fact/1(Roll Rate Fac) -> Product/2
  Constant/1 -> Product/1
  Product1/1 -> Clr/1
  Product/1 -> Clp/1
  wingspan/1 -> roll rate fact/3(wingspan), yaw rate fact/3(wingspan)

== system RefModel_AeroDyn_Sim2/Force and Moment/Aero Surface/Lateral Channel/Cn/yaw factors ==
  p,q,r : Inport
  Airspeed : Inport  Port=2
  wingspan : Inport  Port=3
  Constant : Constant  Value=UAVPARAM_SET.AeroParam.Cn_p
      settings: AttributesFormatString=%<Value>
  Constant1 : Constant  Value=UAVPARAM_SET.AeroParam.Cn_r
      settings: AttributesFormatString=%<Value>
  Get p : Selector  InputPortWidth=3  IndexOptions=Index vector (dialog)  Indices=1  OutputSizes=[(-2)]
  Get r : Selector  InputPortWidth=3  IndexOptions=Index vector (dialog)  Indices=3  OutputSizes=[(-2)]
  Product : Product  SaturateOnIntegerOverflow=on  OutDataTypeStr=Inherit: Same as first input
  Product1 : Product  SaturateOnIntegerOverflow=on  OutDataTypeStr=Inherit: Same as first input
  roll rate fact : Subsystem
  yaw rate fact : Subsystem  AncestorBlock=mbdriLib/Utilities/yaw rate fact
  Cnp : Outport  VectorParamsAs1DForOutWhenUnconnected=off
  Cnr : Outport  Port=2  VectorParamsAs1DForOutWhenUnconnected=off
  wires:
  Airspeed/1 -> yaw rate fact/2(Airspeed), roll rate fact/2(Airspeed)
  Get r/1 -> yaw rate fact/1(r)
  p,q,r/1 -> Get r/1, Get p/1
  Get p/1 -> roll rate fact/1(p)
  roll rate fact/1(Roll Rate Fac) -> Product/2
  Constant/1 -> Product/1
  yaw rate fact/1(Yaw Rate Fac) -> Product1/2
  Constant1/1 -> Product1/1
  Product1/1 -> Cnr/1
  Product/1 -> Cnp/1
  wingspan/1 -> yaw rate fact/3(wingspan), roll rate fact/3(wingspan)

== system RefModel_AeroDyn_Sim2/Force and Moment/Aero Surface/Lateral Channel/Cl/roll factors/roll rate fact ==
  p : Inport
  Airspeed : Inport  Port=2
  wingspan : Inport  Port=3
  Cmq1 : Constant  Value=.5
      settings: AttributesFormatString=%<Value>
  Product : Product  Inputs=***/  SaturateOnIntegerOverflow=on  OutDataTypeStr=Inherit: Same as first input
  Saturation : Saturate  UpperLimit=inf  LowerLimit=0.1
      settings: AttributesFormatString="[%<LowerLimit>  %<UpperLimit>]"
  Roll Rate Fac : Outport  VectorParamsAs1DForOutWhenUnconnected=off
  wires:
  Saturation/1 -> Product/4
  Airspeed/1 -> Saturation/1
  wingspan/1 -> Product/3
  Cmq1/1 -> Product/2
  p/1 -> Product/1
  Product/1 -> Roll Rate Fac/1

== system RefModel_AeroDyn_Sim2/Force and Moment/Aero Surface/Lateral Channel/Cl/roll factors/yaw rate fact ==
  r : Inport
  Airspeed : Inport  Port=2
  wingspan : Inport  Port=3
  Cmq3 : Constant  Value=.5
      settings: AttributesFormatString=%<Value>
  Product1 : Product  Inputs=***/  SaturateOnIntegerOverflow=on  OutDataTypeStr=Inherit: Same as first input
  Saturation : Saturate  UpperLimit=inf  LowerLimit=0.1
      settings: AttributesFormatString="[%<LowerLimit>  %<UpperLimit>]"
  Yaw Rate Fac : Outport  VectorParamsAs1DForOutWhenUnconnected=off
  wires:
  Product1/1 -> Yaw Rate Fac/1
  r/1 -> Product1/1
  Cmq3/1 -> Product1/2
  wingspan/1 -> Product1/3
  Airspeed/1 -> Saturation/1
  Saturation/1 -> Product1/4

== system RefModel_AeroDyn_Sim2/Force and Moment/Aero Surface/Lateral Channel/Cn/yaw factors/roll rate fact ==
  p : Inport
  Airspeed : Inport  Port=2
  wingspan : Inport  Port=3
  Cmq1 : Constant  Value=.5
      settings: AttributesFormatString=%<Value>
  Product : Product  Inputs=***/  SaturateOnIntegerOverflow=on  OutDataTypeStr=Inherit: Same as first input
  Saturation : Saturate  UpperLimit=inf  LowerLimit=0.1
      settings: AttributesFormatString="[%<LowerLimit>  %<UpperLimit>]"
  Roll Rate Fac : Outport  VectorParamsAs1DForOutWhenUnconnected=off
  wires:
  Saturation/1 -> Product/4
  Airspeed/1 -> Saturation/1
  wingspan/1 -> Product/3
  Cmq1/1 -> Product/2
  p/1 -> Product/1
  Product/1 -> Roll Rate Fac/1

== system RefModel_AeroDyn_Sim2/Force and Moment/Aero Surface/Lateral Channel/Cn/yaw factors/yaw rate fact ==
  r : Inport
  Airspeed : Inport  Port=2
  wingspan : Inport  Port=3
  Cmq3 : Constant  Value=.5
      settings: AttributesFormatString=%<Value>
  Product1 : Product  Inputs=***/  SaturateOnIntegerOverflow=on  OutDataTypeStr=Inherit: Same as first input
  Saturation : Saturate  UpperLimit=inf  LowerLimit=0.1
      settings: AttributesFormatString="[%<LowerLimit>  %<UpperLimit>]"
  Yaw Rate Fac : Outport  VectorParamsAs1DForOutWhenUnconnected=off
  wires:
  Product1/1 -> Yaw Rate Fac/1
  r/1 -> Product1/1
  Cmq3/1 -> Product1/2
  wingspan/1 -> Product1/3
  Airspeed/1 -> Saturation/1
  Saturation/1 -> Product1/4

== matlab function RefModel_AeroDyn_Sim2/Force and Moment/Rotor Force/Right Forward/MATLAB Function ==
  data: sideAngle input; forceBody output; lonAngle input; vec0 input
function forceBody = fcn(sideAngle,lonAngle,vec0)
My = [cos(lonAngle) 0 -sin(lonAngle);
      0             1              0;
      sin(lonAngle) 0  cos(lonAngle);];
Mz = [cos(sideAngle)   sin(sideAngle)  0;
     -sin(sideAngle)   cos(sideAngle)  0;
                   0               0   1;];
forceBody = (Mz*My)'*vec0;

== matlab function RefModel_AeroDyn_Sim2/Force and Moment/Rotor Force/Left Forward/MATLAB Function ==
  data: sideAngle input; forceBody output; lonAngle input; vec0 input
function forceBody = fcn(sideAngle,lonAngle,vec0)
My = [cos(lonAngle) 0 -sin(lonAngle);
      0             1              0;
      sin(lonAngle) 0  cos(lonAngle);];
Mz = [cos(sideAngle)   sin(sideAngle)  0;
     -sin(sideAngle)   cos(sideAngle)  0;
                   0               0   1;];
forceBody = (Mz*My)'*vec0;

== matlab function RefModel_AeroDyn_Sim2/Force and Moment/Rotor Force/Right Back/MATLAB Function ==
  data: sideAngle input; forceBody output; lonAngle input; vec0 input
function forceBody = fcn(sideAngle,lonAngle,vec0)
My = [cos(lonAngle) 0 -sin(lonAngle);
      0             1              0;
      sin(lonAngle) 0  cos(lonAngle);];
Mz = [cos(sideAngle)   sin(sideAngle)  0;
     -sin(sideAngle)   cos(sideAngle)  0;
                   0               0   1;];
forceBody = (Mz*My)'*vec0;

== matlab function RefModel_AeroDyn_Sim2/Force and Moment/Rotor Force/Left Back/MATLAB Function ==
  data: sideAngle input; forceBody output; lonAngle input; vec0 input
function forceBody = fcn(sideAngle,lonAngle,vec0)
My = [cos(lonAngle) 0 -sin(lonAngle);
      0             1              0;
      sin(lonAngle) 0  cos(lonAngle);];
Mz = [cos(sideAngle)   sin(sideAngle)  0;
     -sin(sideAngle)   cos(sideAngle)  0;
                   0               0   1;];
forceBody = (Mz*My)'*vec0;

== matlab function RefModel_AeroDyn_Sim2/Force and Moment/Rotor Force/Left Back/Rotor 2814/MATLAB Function ==
  data: u input; y output; poly input
function y = fcn(u, poly)
vec = [u^2,u,1];
y = dot(vec,poly);

== matlab function RefModel_AeroDyn_Sim2/Sensor Model (noise)/Ublox1/add noise1/MATLAB Function ==
  data: u input; k output
function k = fcn(u)
% 
lat = u(1);
deg2m = 111e3;
k = [cos(lat)/deg2m,1/deg2m,1];

== matlab function RefModel_AeroDyn_Sim2/Sensor Model (noise)/um482/add noise1/MATLAB Function ==
  data: u input; k output
function k = fcn(u)
% 
lat = u(1);
deg2m = 111e3;
k = [cos(lat)/deg2m,1/deg2m,1];

== matlab function RefModel_AeroDyn_Sim2/Force and Moment/Rotor Force/Left Back/Rotor 2814/MATLAB Function1 ==
  data: u input; y output; poly input
function y = fcn(u, poly)
vec = [u^2,u,1];
y = dot(vec,poly);

== matlab function RefModel_AeroDyn_Sim2/Force and Moment/Rotor Force/Right Back/Rotor 2814/MATLAB Function ==
  data: u input; y output; poly input
function y = fcn(u, poly)
vec = [u^2,u,1];
y = dot(vec,poly);

== matlab function RefModel_AeroDyn_Sim2/Force and Moment/Rotor Force/Right Back/Rotor 2814/MATLAB Function1 ==
  data: u input; y output; poly input
function y = fcn(u, poly)
vec = [u^2,u,1];
y = dot(vec,poly);

== matlab function RefModel_AeroDyn_Sim2/Force and Moment/Rotor Force/Left Forward/Rotor 5208/MATLAB Function ==
  data: u input; y output; poly input
function y = fcn(u, poly)
vec = [u^2,u,1];
y = dot(vec,poly);

== matlab function RefModel_AeroDyn_Sim2/Force and Moment/Rotor Force/Left Forward/Rotor 5208/MATLAB Function1 ==
  data: u input; y output; poly input
function y = fcn(u, poly)
vec = [u^2,u,1];
y = dot(vec,poly);

== matlab function RefModel_AeroDyn_Sim2/Force and Moment/Rotor Force/Right Forward/Rotor 5208/MATLAB Function ==
  data: u input; y output; poly input
function y = fcn(u, poly)
vec = [u^2,u,1];
y = dot(vec,poly);

== matlab function RefModel_AeroDyn_Sim2/Force and Moment/Rotor Force/Right Forward/Rotor 5208/MATLAB Function1 ==
  data: u input; y output; poly input
function y = fcn(u, poly)
vec = [u^2,u,1];
y = dot(vec,poly);
